simulink model "inicializarILCadaptable"  (R2023b)
settings: Solver=VariableStepAuto  StartTime=0.0  StopTime=25  RelTol=1e-3
settings Model: Creator=LENOVO  LastModifiedBy=LENOVO

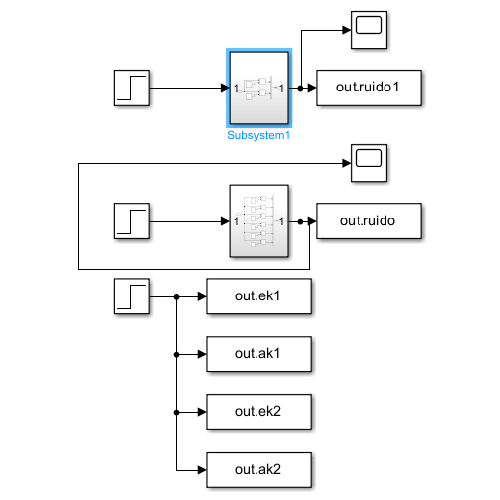
[thumbnail: Simulink's stored preview of the top-level diagram]
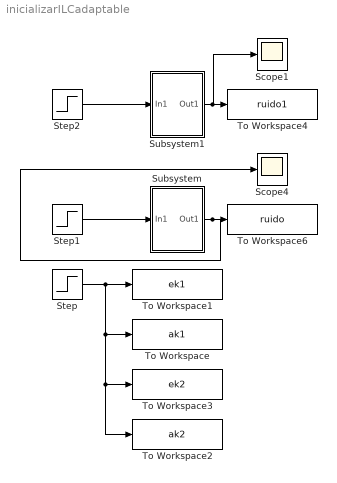
== system inicializarILCadaptable ==
  Scope1 : Scope
  Scope4 : Scope
  Step : Step  After=0  SampleTime=0
  Step1 : Step  Time=0  SampleTime=0
  Step2 : Step  Time=0  SampleTime=0
  Subsystem : Subsystem
  Subsystem1 : Subsystem
  To Workspace : ToWorkspace  VariableName=ak1  SampleTime=-1
  To Workspace1 : ToWorkspace  VariableName=ek1  SampleTime=-1
  To Workspace2 : ToWorkspace  VariableName=ak2  SampleTime=-1
  To Workspace3 : ToWorkspace  VariableName=ek2  SampleTime=-1
  To Workspace4 : ToWorkspace  VariableName=ruido1  SampleTime=-1
  To Workspace6 : ToWorkspace  VariableName=ruido  SampleTime=-1
  wires:
  Step1/1 -> Subsystem/1(In1)
  Subsystem/1(Out1) -> Scope4/1, To Workspace6/1
  Step/1 -> To Workspace2/1, To Workspace3/1, To Workspace/1, To Workspace1/1
  Step2/1 -> Subsystem1/1(In1)
  Subsystem1/1(Out1) -> Scope1/1, To Workspace4/1

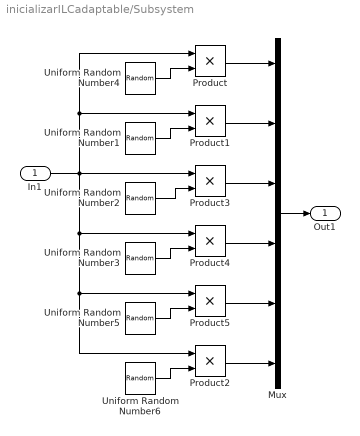
== system inicializarILCadaptable/Subsystem ==
  In1 : Inport
  Mux : Mux  Inputs=6
  Product{,1..5} (6 alike) : Product
  Uniform Random Number1 : UniformRandomNumber  Minimum=-0.0792  Maximum=0.0792  Seed=2  SampleTime=0.1
  Uniform Random Number2 : UniformRandomNumber  Minimum=-0.025  Maximum=0.025  Seed=1  SampleTime=0.1
  Uniform Random Number3 : UniformRandomNumber  Minimum=-0.03  Maximum=0.03  Seed=3  SampleTime=0.1
  Uniform Random Number4 : UniformRandomNumber  Minimum=-0.066  Maximum=0.066  SampleTime=0.1
  Uniform Random Number5 : UniformRandomNumber  Minimum=-0.00138  Maximum=0.00138  Seed=1.5  SampleTime=0.1
  Uniform Random Number6 : UniformRandomNumber  Minimum=-0.00238  Maximum=0.00238  Seed=1.5  SampleTime=0.1
  Out1 : Outport
  wires:
  Product/1 -> Mux/1
  Uniform Random Number5/1 -> Product5/2
  Uniform Random Number1/1 -> Product1/2
  In1/1 -> Product2/1, Product5/1, Product4/1, Product3/1, Product/1, Product1/1
  Uniform Random Number2/1 -> Product3/2
  Product4/1 -> Mux/4
  Product1/1 -> Mux/2
  Uniform Random Number3/1 -> Product4/2
  Uniform Random Number4/1 -> Product/2
  Product3/1 -> Mux/3
  Product5/1 -> Mux/5
  Mux/1 -> Out1/1
  Product2/1 -> Mux/6
  Uniform Random Number6/1 -> Product2/2

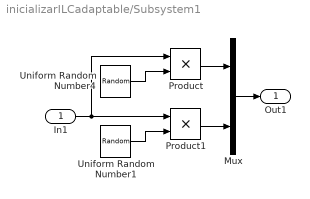
== system inicializarILCadaptable/Subsystem1 ==
  In1 : Inport
  Mux : Mux  Inputs=2
  Product : Product
  Product1 : Product
  Uniform Random Number1 : UniformRandomNumber  Minimum=-0.0792  Maximum=0.0792  Seed=2  SampleTime=0.1
  Uniform Random Number4 : UniformRandomNumber  Minimum=-0.066  Maximum=0.066  SampleTime=0.1
  Out1 : Outport
  wires:
  Product/1 -> Mux/1
  Uniform Random Number1/1 -> Product1/2
  In1/1 -> Product/1, Product1/1
  Product1/1 -> Mux/2
  Uniform Random Number4/1 -> Product/2
  Mux/1 -> Out1/1
